simulink model "FullDynamic"  (R2018a)
settings: Solver=VariableStepAuto  StartTime=0.0  StopTime=10.0  RelTol=1e-3
values from neighbouring files (symbols this model uses):
  B_p = 0.01325    [heli_parameters.m]
  B_y = 0.8513    [heli_parameters.m]
  F_cpp = 1    [heli_parameters.m]
  F_cpy = 1    [heli_parameters.m]
  F_cyp = 1    [heli_parameters.m]
  F_cyy = 1    [heli_parameters.m]
  g = 9.81    [Spoustec_simu.m]    (also in heli_parameters.m)
  h = 0.00714    [Spoustec_simu.m]    (also in heli_parameters.m)
  J_eqp = 0.0332    [heli_parameters.m]
  J_eqy = 0.0371    [heli_parameters.m]
  K_pp = 0.02638    [heli_parameters.m]
  K_py = 0.00189    [heli_parameters.m]
  K_yp = 0.002096    [heli_parameters.m]
  K_yy = 0.01871    [heli_parameters.m]
  l_mc = 0.0122    [heli_parameters.m]
  m = 1.3872    [Spoustec_simu.m]    (also in heli_parameters.m)
settings Model: Creator=ja  LastModifiedBy=ja

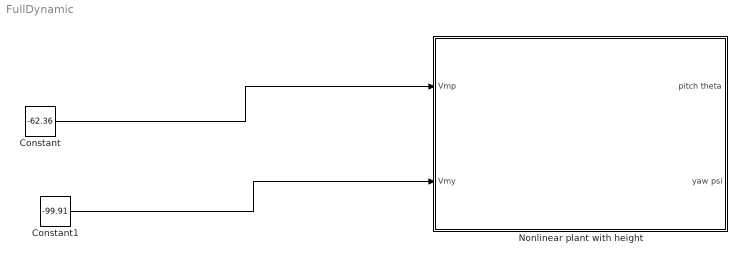
== system FullDynamic ==
  Constant : Constant  Value=-62.36
  Constant1 : Constant  Value=-99.91
  Nonlinear plant with height : Subsystem
      mask Display: image('Dynamics-of-2DOF-Helicopter.png');
  wires:
  Constant1/1 -> Nonlinear plant with height/2("Vmy ")
  Constant/1 -> Nonlinear plant with height/1("Vmp ")

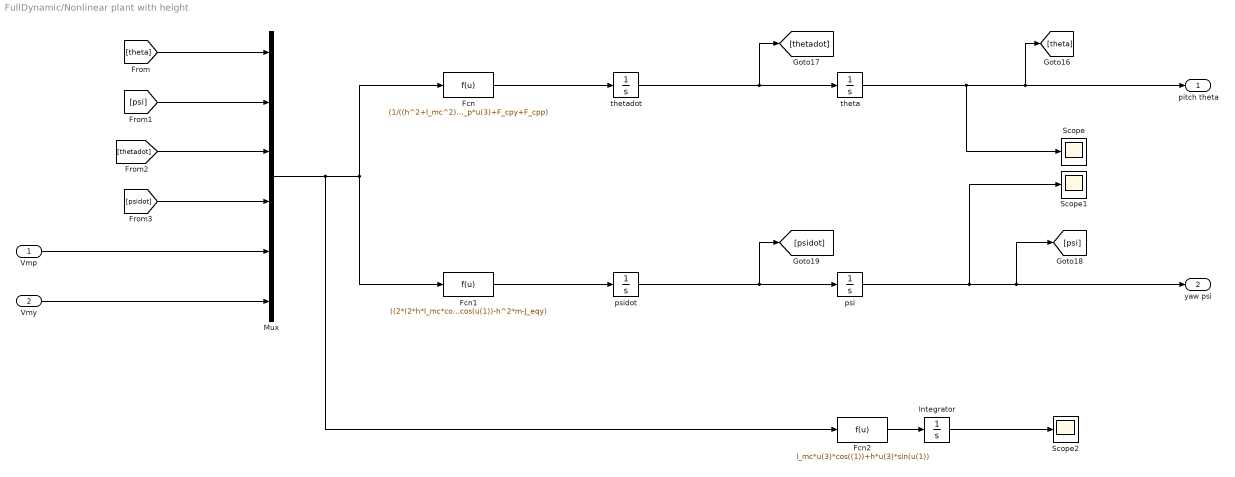
== system FullDynamic/Nonlinear plant with height ==
  "Vmp " : Inport
  "Vmy " : Inport  Port=2
  Fcn : Fcn  Expr=(1/((h^2+l_mc^2)*m+J_eqp))*(2*m*(h*l_mc*cos(u(1))^2+sin(u(1))*(h^2/2-l_mc^2/2)*cos(u(1))-(h*l_mc)/2)*u(4)^2-cos(u(1))*g*l_mc*m-sin(u(1))*g*h*m+K_pp*u(5)+K_py*u(6)-B_p*u(3)+F_cpy+F_cpp)
  Fcn1 : Fcn  Expr=((2*(2*h*l_mc*cos(u(1))^2+sin(u(1))*(h^2-l_mc^2)*cos(u(1))-h*l_mc)*m*u(3)+B_y)*u(4)-cos(u(1))*(K_yy*u(6)+K_yp*u(5)+F_cyp+F_cyy))/(m*(h^2-l_mc^2)*cos(u(1))^2-2*sin(u(1))*h*m*l_mc*cos(u(1))-h^2*m-J_eqy)
  Fcn2 : Fcn  Expr=l_mc*u(3)*cos((1))+h*u(3)*sin(u(1))
  Integrator : Integrator
  Mux : Mux  Inputs=6
  Scope : Scope
  Scope1 : Scope
  Scope2 : Scope
  psi : Integrator
  psidot : Integrator
  theta : Integrator
  thetadot : Integrator
  pitch theta : Outport
  "yaw psi " : Outport  Port=2
  wires:
  [psi] -> Mux/2
  Fcn/1 -> thetadot/1
  "Vmp "/1 -> Mux/5
  Mux/1 -> Fcn2/1, Fcn1/1, Fcn/1
  [thetadot] -> Mux/3
  psidot/1 -> [psidot], psi/1
  psi/1 -> Scope1/1, "yaw psi "/1, [psi]
  Fcn1/1 -> psidot/1
  "Vmy "/1 -> Mux/6
  [theta] -> Mux/1
  thetadot/1 -> [thetadot], theta/1
  theta/1 -> Scope/1, pitch theta/1, [theta]
  [psidot] -> Mux/4
  Fcn2/1 -> Integrator/1
  Integrator/1 -> Scope2/1
